simulink model "exemplo_bloco_modelo"  (R2015a)
settings: Solver=ode45  SolverMode=SingleTasking  StartTime=0.0  StopTime=10  FixedStep=0.0005  RelTol=1e-6
undefined symbols (not defined in the file): magnitude
settings Model: CovSFcnEnable=off  Creator=Mauricio  LastModifiedBy=YecidMoreno
settings OptimizationCC: InitFltsAndDblsToZero=on
settings DebuggingCC: SaveWithParameterizedLinksMsg=none  SignalResolutionControl=TryResolveAllWithWarning  SolverPrmCheckMsg=warning  MultiTaskDSMMsg=warning  MultiTaskCondExecSysMsg=none  FcnCallInpInsideContextMsg=UseLocalSettings
settings GRTTargetCC: TargetFcnLib=ansi_tfl_tmw.mat  CombineOutputUpdateFcns=off  GRTInterface=on

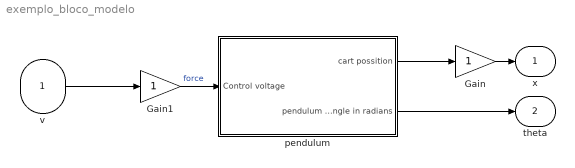
== system exemplo_bloco_modelo ==
  v : Inport
  Gain : Gain
  Gain1 : Gain
  pendulum : Subsystem  mask{m=0.23, cM=2.4, L=0.4, g=9.81, I=0.099, theta0=0.2, cart_friction=0.05, pend_damp=0.005}
      mask prompts: m "Pendulum mass"; cM "Cart mass"; L "Pendulum length"; g "gravitational constant"; I "Moment of inertia of the pole itself"; theta0 "Initial pendulum angle"; cart_friction "Cart friction coefficient"; pend_damp "Pendulum damping coefficient"
  x : Outport
  theta : Outport  Port=2
  wires:
  Gain1/1 -> pendulum/1(Control voltage)  "force"
  pendulum/1(cart possition) -> Gain/1
  v/1 -> Gain1/1
  Gain/1 -> x/1
  pendulum/2(pendulum angle in radians) -> theta/1

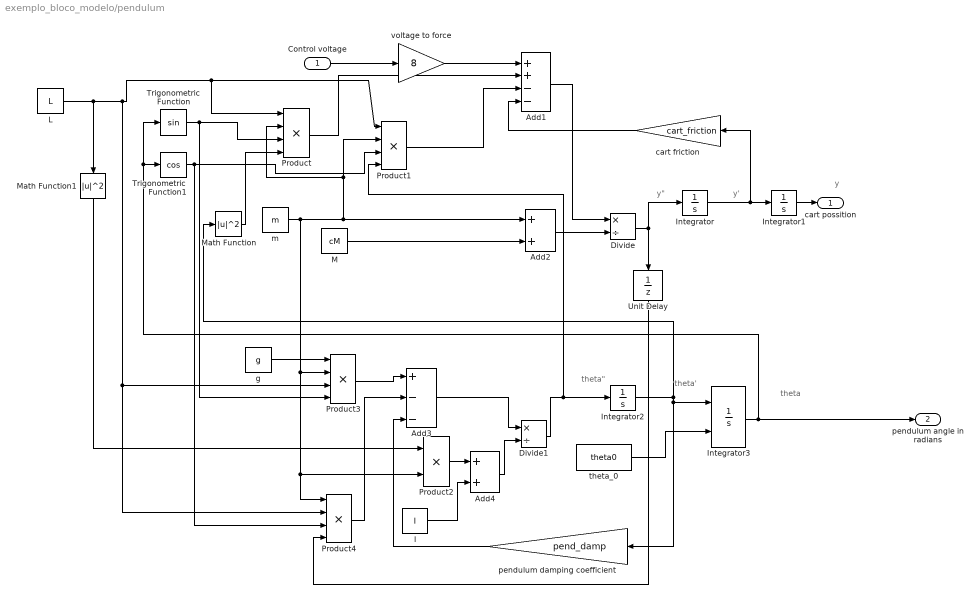
== system exemplo_bloco_modelo/pendulum ==
  note: y
  note: theta
  note: theta'
  note: theta"
  note: y'
  note: y"
  Control voltage : Inport
  Add1 : Sum  Inputs=++--
  Add2 : Sum
  Add3 : Sum  Inputs=+--
  Add4 : Sum
  Divide : Product  Inputs=*/
  Divide1 : Product  Inputs=*/
  I : Constant  Value=I
  Integrator : Integrator
  Integrator1 : Integrator
  Integrator2 : Integrator
  Integrator3 : Integrator  InitialConditionSource=external
  L : Constant  Value=L
  M : Constant  Value=cM
  Math Function : Math  Operator=magnitude^2  SaturateOnIntegerOverflow=on
  Math Function1 : Math  Operator=magnitude^2  SaturateOnIntegerOverflow=on
  Product{,1,3..4} (4 alike) : Product  Inputs=4  RndMeth=Zero
  Product2 : Product  RndMeth=Zero
  Trigonometric Function : Trigonometry
  Trigonometric Function1 : Trigonometry  Operator=cos
  Unit Delay : UnitDelay  SampleTime=0.001
  cart friction : Gain  Gain=cart_friction
  g : Constant  Value=g
  m : Constant  Value=m
  pendulum damping coefficient : Gain  Gain=pend_damp
  theta_0 : Constant  Value=theta0
  voltage to force : Gain  Gain=8
  cart possition : Outport
  pendulum angle in radians : Outport  Port=2
  wires:
  Integrator/1 -> Integrator1/1, cart friction/1
  Integrator2/1 -> Integrator3/1, pendulum damping coefficient/1, Math Function/1
  Integrator3/1 -> Trigonometric Function1/1, Trigonometric Function/1, pendulum angle in radians/1
  m/1 -> Add2/1, Product/2, Product1/2, Product3/2, Product2/2, Product4/1
  M/1 -> Add2/2
  Add2/1 -> Divide/2
  Add1/1 -> Divide/1
  Divide/1 -> Integrator/1, Unit Delay/1
  Divide1/1 -> Integrator2/1, Product1/4
  L/1 -> Math Function1/1, Product/1, Product1/1, Product3/3, Product4/2
  Trigonometric Function/1 -> Product/3, Product3/4
  theta_0/1 -> Integrator3/2
  Math Function/1 -> Product/4
  Product/1 -> Add1/2
  Product1/1 -> Add1/3
  Trigonometric Function1/1 -> Product1/3, Product4/3
  Add3/1 -> Divide1/1
  Math Function1/1 -> Product2/1
  Product3/1 -> Add3/1
  Product4/1 -> Add3/2
  g/1 -> Product3/1
  cart friction/1 -> Add1/4
  pendulum damping coefficient/1 -> Add3/3
  Integrator1/1 -> cart possition/1
  Product2/1 -> Add4/1
  Add4/1 -> Divide1/2
  I/1 -> Add4/2
  Unit Delay/1 -> Product4/4
  Control voltage/1 -> voltage to force/1
  voltage to force/1 -> Add1/1
